simulink model "powerwindow_cv"  (Simulink 7.6)
settings: Solver=FixedStepDiscrete  StartTime=0.0  StopTime=inf  FixedStep=1e-4  RelTol=1e-3
libraries: simulink x6
settings Model: Creator=The MathWorks Inc.  ExtModeAutoUpdateStatusClock=off
settings DataIOCC: SignalLoggingName=sigsOut
settings OptimizationCC: BooleanDataType=off  InitFltsAndDblsToZero=on
settings DebuggingCC: SaveWithParameterizedLinksMsg=none  SignalResolutionControl=TryResolveAllWithWarning  SolverPrmCheckMsg=none  MultiTaskDSMMsg=warning  MultiTaskCondExecSysMsg=none
settings HardwareCC: ProdHWDeviceType=Specified
settings SFSimCC: SimParseCustomCode=off
settings RTWCC: IncludeERTFirstTime=on
settings CodeAppCC: CustomSymbolStrFcn=$F$N$M
settings GRTTargetCC: TargetFcnLib=ansi_tfl_tmw.mat

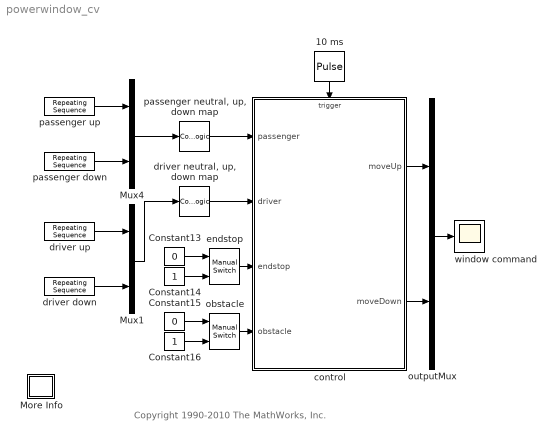
== system powerwindow_cv ==
  note: Copyright 1990-2010 The MathWorks, Inc.
  10 ms : DiscretePulseGenerator  PulseType=Time based  Period=1e-2  PulseWidth=50  SampleTime=1e-3
  Constant13 : Constant  Value=0
  Constant14 : Constant
  Constant15 : Constant  Value=0
  Constant16 : Constant
  More Info : Subsystem
      settings: OpenFcn=showdemo(bdroot(gcb))
      mask Display: disp('?')
  Mux1 : Mux  Inputs=2
  Mux4 : Mux  Inputs=2
  control : Stateflow chart  TreatAsAtomicUnit=on
  "driver neutral, up, down map" : CombinatorialLogic  TruthTable=[1 0 0;0 0 1;0 1 0;1 0 0]
  driver down : simulink/Sources/Repeating Sequence  SystemSampleTime=-1  rep_seq_t=[0 1 2 3 4 5 6]  rep_seq_y=[0 1 0 0 1 1 0]
  driver up : simulink/Sources/Repeating Sequence  SystemSampleTime=-1  rep_seq_t=[0 1 2 3 4 5 6]  rep_seq_y=[0 0 1 0 1 0 1]
  endstop : simulink/Signal Routing/Manual Switch  SystemSampleTime=-1  sw=1  action=0  varsize=off
  obstacle : simulink/Signal Routing/Manual Switch  SystemSampleTime=-1  sw=1  action=0  varsize=off
  outputMux : Mux  Inputs=2
  "passenger neutral, up, down map" : CombinatorialLogic  TruthTable=[1 0 0;0 0 1;0 1 0;1 0 0]
  passenger down : simulink/Sources/Repeating Sequence  SystemSampleTime=-1  rep_seq_t=[0 1 2 3 4 5 6]  rep_seq_y=[0 0 0 1 0 1 1]
  passenger up : simulink/Sources/Repeating Sequence  SystemSampleTime=-1  rep_seq_t=[0 1 2 3 4 5 6]  rep_seq_y=[0 0 0 0 0 0 0]
  window command : Scope
      settings: YMin=0  YMax=1
  wires:
  10 ms/1 -> control/Trigger
  passenger down/1 -> Mux4/2
  driver down/1 -> Mux1/2
  Mux4/1 -> "passenger neutral, up, down map"/1
  Mux1/1 -> "driver neutral, up, down map"/1
  "passenger neutral, up, down map"/1 -> control/1(passenger)
  "driver neutral, up, down map"/1 -> control/2(driver)
  passenger up/1 -> Mux4/1
  driver up/1 -> Mux1/1
  control/1(moveUp) -> outputMux/1
  control/2(moveDown) -> outputMux/2
  outputMux/1 -> window command/1
  Constant13/1 -> endstop/1
  Constant14/1 -> endstop/2
  Constant15/1 -> obstacle/1
  Constant16/1 -> obstacle/2
  endstop/1 -> control/3(endstop)
  obstacle/1 -> control/4(obstacle)

== system powerwindow_cv/More Info ==

== stateflow chart control ==
  settings: executeAtInitialization=1
  state emergencyDown
    entry:
    moveUp = 0;
    moveDown = 1;
  state safe
    state driverUp
      entry: moveUp = 1;
      exit: moveUp = 0;
      state iniDriverUp
      state DriverUp
      state autoDriverUp
      iniDriverUp -> (junction 26) : after(100,ticks)
      (junction 26) -> DriverUp [order 2]
      (junction 26) -> autoDriverUp [order 1] : [driver[1]]
    state driverDown
      entry: moveDown = 1;
      exit: moveDown = 0;
      state iniDriverDown
      state DriverDown
      state autoDriverDown
      iniDriverDown -> (junction 25) : after(100,ticks)
      (junction 25) -> autoDriverDown [order 1] : [driver[1]]
      (junction 25) -> DriverDown [order 2]
    state driverNeutral
      entry:
      moveUp = 0;
      moveDown = 0;
      state passengerneutral
        entry:
        moveUp = 0;
        moveDown = 0;
      state passengerUp
        entry: moveUp = 1;
        exit: moveUp = 0;
        state iniPassengerUp
        state PassengerUp
        state autoPassengerUp
        (junction 24) -> PassengerUp [order 2]
        (junction 24) -> autoPassengerUp [order 1] : [passenger[1]]
        iniPassengerUp -> (junction 24) : after(100,ticks)
      state passengerDown
        entry: moveDown = 1;
        exit: moveDown = 0;
        state iniPassengerDown
        state passengerDown
        state autoPassengerDown
        (junction 23) -> autoPassengerDown [order 1] : [passenger[1]]
        iniPassengerDown -> (junction 23) : after(100,ticks)
        (junction 23) -> safe.driverNeutral.passengerDown.passengerDown [order 2]
      safe.driverNeutral.passengerDown.passengerDown -> passengerneutral : [passenger[1]]
      safe.driverNeutral.passengerDown -> passengerneutral [order 1] : [endstop]
      PassengerUp -> passengerneutral : [passenger[1]]
      passengerUp -> passengerneutral [order 2] : [endstop]
      passengerneutral -> iniPassengerDown [order 2] : [passenger[3]]
      passengerneutral -> iniPassengerUp [order 1] : [passenger[2]]
      safe.driverNeutral.passengerDown -> PassengerUp [order 2] : [passenger[2]]
      passengerUp -> safe.driverNeutral.passengerDown.passengerDown [order 1] : [passenger[3]]
      (default) -> passengerneutral
    driverNeutral -> iniDriverDown [order 2] : [driver[3]]
    driverUp -> DriverDown [order 1] : [driver[3]]
    driverDown -> DriverUp [order 2] : [driver[2]]
    driverNeutral -> iniDriverUp [order 1] : [driver[2]]
    DriverDown -> driverNeutral : [driver[1]]
    DriverUp -> driverNeutral : [driver[1]]
    driverDown -> driverNeutral [order 1] : [endstop]
    driverUp -> driverNeutral [order 2] : [endstop]
    (default) -> driverNeutral
  emergencyDown -> passengerneutral : [endstop | after(100,ticks)]
  safe -> emergencyDown : [obstacle]
  (default) -> safe
  data: passenger input boolean size=3; driver input boolean size=3; moveUp output double; moveDown output double; endstop input double; obstacle input double
  events: ticks input RISING_EDGE_EVENT
